simulink model "friction_rt_online_generated"  (R2025a)
settings: Solver=VariableStepAuto  StartTime=0.0  StopTime=100  RelTol=1e-3
settings Model: Creator=Kylo_Ren  LastModifiedBy=Kylo_Ren

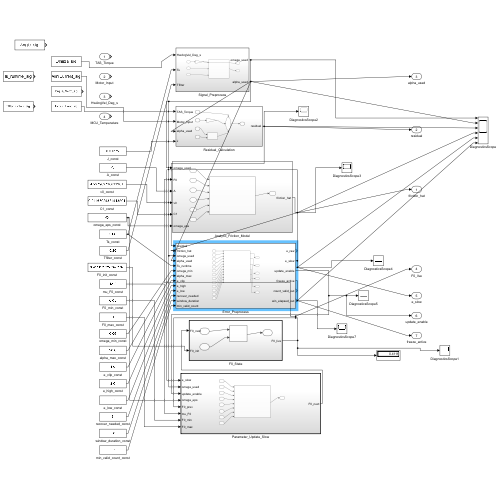
[thumbnail: Simulink's stored preview of the top-level diagram]
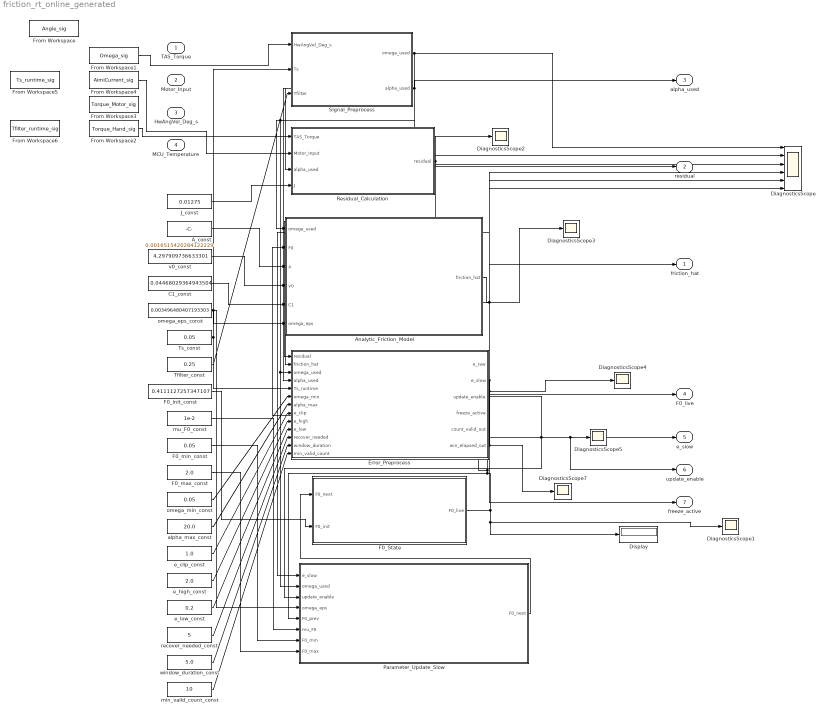
== system friction_rt_online_generated ==
  TAS_Torque : Inport
  Motor_Input : Inport  Port=2
  HwAngVel_Deg_s : Inport  Port=3
  MCU_Temperature : Inport  Port=4
  A_const : Constant  Value=0.0016515420284122229
  Analytic_Friction_Model : Subsystem
  C1_const : Constant  Value=0.04468029364943504
  DiagnosticsScope : Scope  NumInputPorts=6
  DiagnosticsScope{1..5,7} (6 alike) : Scope
      DiagnosticsScope1 settings: ActiveDisplayYMinimum=0.31111272573471072  ActiveDisplayYMaximum=0.51111272573471067
      DiagnosticsScope2 settings: ActiveDisplayYMinimum=-1.2927992978331837  ActiveDisplayYMaximum=1.3052950610427259
      DiagnosticsScope3 settings: ActiveDisplayYMinimum=-0.552517030526273  ActiveDisplayYMaximum=0.552517030526273
      DiagnosticsScope4 settings: ActiveDisplayYMinimum=-1  ActiveDisplayYMaximum=1
      DiagnosticsScope5 settings: ActiveDisplayYMinimum=-1  ActiveDisplayYMaximum=1
      DiagnosticsScope7 settings: ActiveDisplayYMinimum=-1  ActiveDisplayYMaximum=1
  Display : Display
  Error_Preprocess : Subsystem
  F0_State : Subsystem  TreatAsAtomicUnit=on
  F0_init_const : Constant  Value=0.4111127257347107
  F0_max_const : Constant  Value=2.0
  F0_min_const : Constant  Value=0.05
  From Workspace : FromWorkspace  VariableName=Angle_sig
  From Workspace1 : FromWorkspace  VariableName=Omega_sig
  From Workspace2 : FromWorkspace  VariableName=Torque_Hand_sig
  From Workspace3 : FromWorkspace  VariableName=Torque_Motor_sig
  From Workspace4 : FromWorkspace  VariableName=AimiCurrent_sig
  From Workspace5 : FromWorkspace  VariableName=Ts_runtime_sig
  From Workspace6 : FromWorkspace  VariableName=Tfilter_runtime_sig
  J_const : Constant  Value=0.01275
  Parameter_Update_Slow : Subsystem  TreatAsAtomicUnit=on
  Residual_Calculation : Subsystem
  Signal_Preprocess : Subsystem
  Tfilter_const : Constant  Value=0.25
  Ts_const : Constant  Value=0.05
  alpha_max_const : Constant  Value=20.0
  e_clip_const : Constant  Value=1.0
  e_high_const : Constant  Value=2.0
  e_low_const : Constant  Value=0.2
  min_valid_count_const : Constant  Value=10
  mu_F0_const : Constant  Value=1e-2
  omega_eps_const : Constant  Value=0.003496480407193303
  omega_min_const : Constant  Value=0.05
  recover_needed_const : Constant  Value=5
  v0_const : Constant  Value=4.297909736633301
  window_duration_const : Constant  Value=5.0
  friction_hat : Outport
  residual : Outport  Port=2
  alpha_used : Outport  Port=3
  F0_live : Outport  Port=4
  e_slow : Outport  Port=5
  update_enable : Outport  Port=6
  freeze_active : Outport  Port=7
  wires:
  From Workspace1/1 -> Signal_Preprocess/1(HwAngVel_Deg_s)
  Ts_const/1 -> Signal_Preprocess/2(Ts), Error_Preprocess/5(Ts_runtime)
  Tfilter_const/1 -> Signal_Preprocess/3(Tfilter)
  Signal_Preprocess/1(omega_used) -> Error_Preprocess/3(omega_used), Parameter_Update_Slow/2(omega_used), Analytic_Friction_Model/1(omega_used), DiagnosticsScope/1
  Signal_Preprocess/2(alpha_used) -> Residual_Calculation/3(alpha_used), Error_Preprocess/4(alpha_used), alpha_used/1, DiagnosticsScope/2
  From Workspace2/1 -> Residual_Calculation/1(TAS_Torque)
  From Workspace4/1 -> Residual_Calculation/2(Motor_Input)
  J_const/1 -> Residual_Calculation/4(J)
  Residual_Calculation/1(residual) -> Error_Preprocess/1(residual), residual/1, DiagnosticsScope/3, DiagnosticsScope2/1
  Analytic_Friction_Model/1(friction_hat) -> Error_Preprocess/2(friction_hat), friction_hat/1, DiagnosticsScope/4, DiagnosticsScope3/1
  omega_min_const/1 -> Error_Preprocess/6(omega_min)
  alpha_max_const/1 -> Error_Preprocess/7(alpha_max)
  e_clip_const/1 -> Error_Preprocess/8(e_clip)
  e_high_const/1 -> Error_Preprocess/9(e_high)
  e_low_const/1 -> Error_Preprocess/10(e_low)
  recover_needed_const/1 -> Error_Preprocess/11(recover_needed)
  window_duration_const/1 -> Error_Preprocess/12(window_duration)
  min_valid_count_const/1 -> Error_Preprocess/13(min_valid_count)
  Error_Preprocess/2(e_slow) -> e_slow/1, DiagnosticsScope/5, DiagnosticsScope4/1, Parameter_Update_Slow/1(e_slow)
  Error_Preprocess/3(update_enable) -> update_enable/1, DiagnosticsScope5/1, Parameter_Update_Slow/3(update_enable)
  omega_eps_const/1 -> Parameter_Update_Slow/4(omega_eps), Analytic_Friction_Model/6(omega_eps)
  F0_State/1(F0_live) -> DiagnosticsScope1/1, Display/1, Parameter_Update_Slow/5(F0_prev), Analytic_Friction_Model/2(F0), F0_live/1
  mu_F0_const/1 -> Parameter_Update_Slow/6(mu_F0)
  F0_min_const/1 -> Parameter_Update_Slow/7(F0_min)
  F0_max_const/1 -> Parameter_Update_Slow/8(F0_max)
  Parameter_Update_Slow/1(F0_next) -> F0_State/1(F0_next)
  F0_init_const/1 -> F0_State/2(F0_init)
  A_const/1 -> Analytic_Friction_Model/3(A)
  v0_const/1 -> Analytic_Friction_Model/4(v0)
  C1_const/1 -> Analytic_Friction_Model/5(C1)
  Error_Preprocess/4(freeze_active) -> freeze_active/1, DiagnosticsScope/6, DiagnosticsScope7/1

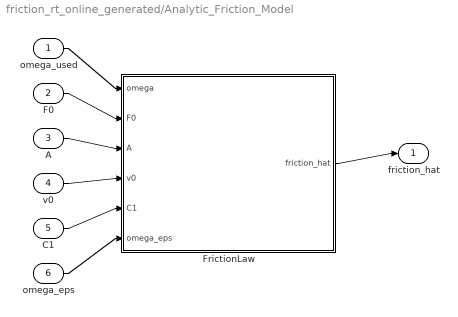
== system friction_rt_online_generated/Analytic_Friction_Model ==
  omega_used : Inport
  F0 : Inport  Port=2
  A : Inport  Port=3
  v0 : Inport  Port=4
  C1 : Inport  Port=5
  omega_eps : Inport  Port=6
  FrictionLaw : MATLAB Function  TreatAsAtomicUnit=on
  friction_hat : Outport
  wires:
  omega_used/1 -> FrictionLaw/1(omega)
  F0/1 -> FrictionLaw/2(F0)
  A/1 -> FrictionLaw/3(A)
  v0/1 -> FrictionLaw/4(v0)
  C1/1 -> FrictionLaw/5(C1)
  omega_eps/1 -> FrictionLaw/6(omega_eps)
  FrictionLaw/1(friction_hat) -> friction_hat/1

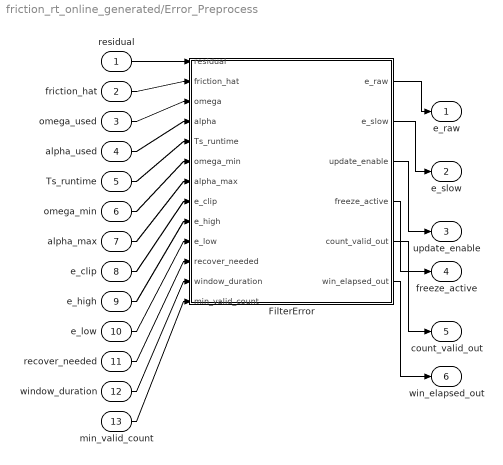
== system friction_rt_online_generated/Error_Preprocess ==
  residual : Inport
  friction_hat : Inport  Port=2
  omega_used : Inport  Port=3
  alpha_used : Inport  Port=4
  Ts_runtime : Inport  Port=5
  omega_min : Inport  Port=6
  alpha_max : Inport  Port=7
  e_clip : Inport  Port=8
  e_high : Inport  Port=9
  e_low : Inport  Port=10
  recover_needed : Inport  Port=11
  window_duration : Inport  Port=12
  min_valid_count : Inport  Port=13
  FilterError : MATLAB Function  TreatAsAtomicUnit=on
  e_raw : Outport
  e_slow : Outport  Port=2
  update_enable : Outport  Port=3
  freeze_active : Outport  Port=4
  count_valid_out : Outport  Port=5
  win_elapsed_out : Outport  Port=6
  wires:
  residual/1 -> FilterError/1(residual)
  friction_hat/1 -> FilterError/2(friction_hat)
  omega_used/1 -> FilterError/3(omega)
  alpha_used/1 -> FilterError/4(alpha)
  Ts_runtime/1 -> FilterError/5(Ts_runtime)
  omega_min/1 -> FilterError/6(omega_min)
  alpha_max/1 -> FilterError/7(alpha_max)
  e_clip/1 -> FilterError/8(e_clip)
  e_high/1 -> FilterError/9(e_high)
  e_low/1 -> FilterError/10(e_low)
  recover_needed/1 -> FilterError/11(recover_needed)
  window_duration/1 -> FilterError/12(window_duration)
  min_valid_count/1 -> FilterError/13(min_valid_count)
  FilterError/1(e_raw) -> e_raw/1
  FilterError/2(e_slow) -> e_slow/1
  FilterError/3(update_enable) -> update_enable/1
  FilterError/4(freeze_active) -> freeze_active/1
  FilterError/5(count_valid_out) -> count_valid_out/1
  FilterError/6(win_elapsed_out) -> win_elapsed_out/1

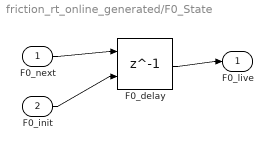
== system friction_rt_online_generated/F0_State ==
  F0_next : Inport
  F0_init : Inport  Port=2
  F0_delay : Delay  DelayLength=1  InitialConditionSource=Input port
      settings: InputPortMap=u0,p4
  F0_live : Outport
  wires:
  F0_next/1 -> F0_delay/1
  F0_init/1 -> F0_delay/2
  F0_delay/1 -> F0_live/1

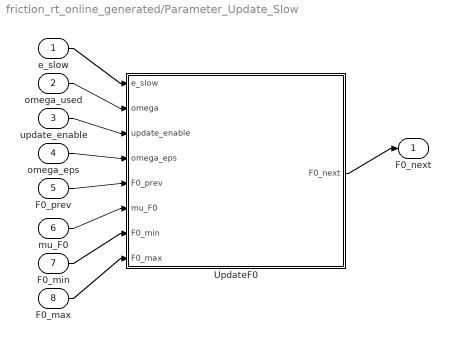
== system friction_rt_online_generated/Parameter_Update_Slow ==
  e_slow : Inport
  omega_used : Inport  Port=2
  update_enable : Inport  Port=3
  omega_eps : Inport  Port=4
  F0_prev : Inport  Port=5
  mu_F0 : Inport  Port=6
  F0_min : Inport  Port=7
  F0_max : Inport  Port=8
  UpdateF0 : MATLAB Function  TreatAsAtomicUnit=on
  F0_next : Outport
  wires:
  e_slow/1 -> UpdateF0/1(e_slow)
  omega_used/1 -> UpdateF0/2(omega)
  update_enable/1 -> UpdateF0/3(update_enable)
  omega_eps/1 -> UpdateF0/4(omega_eps)
  F0_prev/1 -> UpdateF0/5(F0_prev)
  mu_F0/1 -> UpdateF0/6(mu_F0)
  F0_min/1 -> UpdateF0/7(F0_min)
  F0_max/1 -> UpdateF0/8(F0_max)
  UpdateF0/1(F0_next) -> F0_next/1

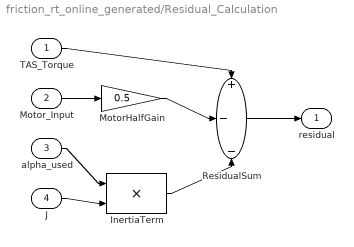
== system friction_rt_online_generated/Residual_Calculation ==
  TAS_Torque : Inport
  Motor_Input : Inport  Port=2
  alpha_used : Inport  Port=3
  J : Inport  Port=4
  InertiaTerm : Product
  MotorHalfGain : Gain  Gain=0.5
  ResidualSum : Sum  Inputs=+--
  residual : Outport
  wires:
  TAS_Torque/1 -> ResidualSum/1
  Motor_Input/1 -> MotorHalfGain/1
  MotorHalfGain/1 -> ResidualSum/2
  alpha_used/1 -> InertiaTerm/1
  J/1 -> InertiaTerm/2
  InertiaTerm/1 -> ResidualSum/3
  ResidualSum/1 -> residual/1

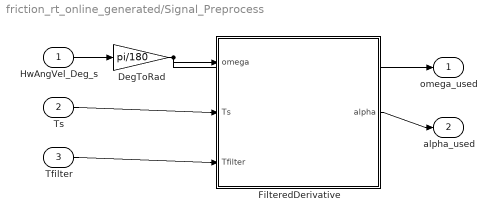
== system friction_rt_online_generated/Signal_Preprocess ==
  HwAngVel_Deg_s : Inport
  Ts : Inport  Port=2
  Tfilter : Inport  Port=3
  DegToRad : Gain  Gain=pi/180
  FilteredDerivative : MATLAB Function  TreatAsAtomicUnit=on
  omega_used : Outport
  alpha_used : Outport  Port=2
  wires:
  HwAngVel_Deg_s/1 -> DegToRad/1
  DegToRad/1 -> FilteredDerivative/1(omega), omega_used/1
  Ts/1 -> FilteredDerivative/2(Ts)
  Tfilter/1 -> FilteredDerivative/3(Tfilter)
  FilteredDerivative/1(alpha) -> alpha_used/1

== matlab function friction_rt_online_generated/Analytic_Friction_Model/FrictionLaw ==
  data: omega input; friction_hat output; F0 input; A input; v0 input; C1 input; omega_eps input
function friction_hat = fcn(omega, F0, A, v0, C1, omega_eps)                             
                                                                                        % Analytic friction law:                                                                 
                                                                                        % friction_hat = tanh(omega/omega_eps) * (F0 + A*(1-exp(-abs(omega)/v0)) + C1*abs(omega))
                                                                                        absw = abs(omega);                                                                       
                                                                                        s = tanh(omega / max(omega_eps, 1e-6));                                                  
                                                                                        phi = 1.0 - exp(-absw / max(v0, 1e-6));                                                  
                                                                                        mag = F0 + A * phi + C1 * absw;                                                          
                                                                                        if mag < 0.0                                                                             
                                                                                            mag = 0.0;                                                                           
                                                                                        end                                                                                      
                                                                                        friction_hat = s * mag;

== matlab function friction_rt_online_generated/Signal_Preprocess/FilteredDerivative ==
  data: omega input; alpha output; Ts input; Tfilter input
function alpha = fcn(omega, Ts, Tfilter)        
                                               % Filtered derivative used for the inertia term.
                                               % X[k] = (Ts/T) * omega[k] + (1 - Ts/T) * X[k-1]
                                               % alpha[k] = (1/T) * (omega[k] - X[k-1])        
                                               persistent x_prev                               
                                               if isempty(x_prev)                              
                                                   x_prev = omega;                             
                                               end                                             
                                               a = Ts / max(Tfilter, 1e-6);                    
                                               a = min(max(a, 0.0), 1.0);                      
                                               alpha = (omega - x_prev) / max(Tfilter, 1e-6);  
                                               x_new = a * omega + (1.0 - a) * x_prev;         
                                               x_prev = x_new;

== matlab function friction_rt_online_generated/Error_Preprocess/FilterError ==
  data: residual input; e_raw output; friction_hat input; omega input; alpha input; Ts_runtime input; omega_min input; alpha_max input; e_clip input; e_high input; e_low input; recover_needed input; window_duration input; min_valid_count input; e_slow output; update_enable output; freeze_active output; count_valid_out output; win_elapsed_out output
function [e_raw, e_slow, update_enable, freeze_active, count_valid_out, win_elapsed_out] = fcn(residual, friction_hat, omega, alpha, Ts_runtime, omega_min, alpha_max, e_clip, e_high, e_low, recover_needed, window_duration, min_valid_count)
    % Build a reliable batch adaptation error.                                                                                                                                                                   
    % 1) compute signed mismatch e_raw for diagnostics                                                                                                                                                           
    % 2) compute magnitude-domain mismatch for F0 adaptation                                                                                                                                                     
    % 3) collect trusted samples in a time window                                                                                                                                                                
    % 4) update only once per window using the window average                                                                                                                                                    
    persistent e_hold freeze_state recover_count win_elapsed sum_mag count_valid                                                                                                                                 
    if isempty(e_hold)                                                                                                                                                                                           
    e_hold = 0.0;                                                                                                                                                                                            
    freeze_state = false;                                                                                                                                                                                    
    recover_count = 0;                                                                                                                                                                                       
    win_elapsed = 0.0;                                                                                                                                                                                       
    sum_mag = 0.0;                                                                                                                                                                                           
    count_valid = 0;                                                                                                                                                                                         
    end                                                                                                                                                                                                          
    e_raw = residual - friction_hat;                                                                                                                                                                             
    e_mag = abs(residual) - abs(friction_hat);                                                                                                                                                                   
    trusted_sample = (abs(omega) > omega_min) && (abs(alpha) < alpha_max);                                                                                                                                       
    anomaly = (abs(e_raw) > e_high) || (abs(alpha) > alpha_max);                                                                                                                                                 
    recovered = trusted_sample && (abs(e_raw) < e_low);                                                                                                                                                          
    if ~freeze_state && anomaly                                                                                                                                                                                  
    freeze_state = true;                                                                                                                                                                                     
    recover_count = 0;                                                                                                                                                                                       
    elseif freeze_state                                                                                                                                                                                          
    if recovered                                                                                                                                                                                             
    recover_count = recover_count + 1;                                                                                                                                                                   
    if recover_count >= recover_needed                                                                                                                                                                   
    freeze_state = false;                                                                                                                                                                            
    recover_count = 0;                                                                                                                                                                               
    end                                                                                                                                                                                                  
    else                                                                                                                                                                                                     
    recover_count = 0;                                                                                                                                                                                   
    end                                                                                                                                                                                                      
    end                                                                                                                                                                                                          
    freeze_active = freeze_state;                                                                                                                                                                                
    sample_ok = trusted_sample && ~freeze_state;                                                                                                                                                                 
    e_used = e_mag;                                                                                                                                                                                              
    if e_used > e_clip                                                                                                                                                                                           
    e_used = e_clip;                                                                                                                                                                                         
    elseif e_used < -e_clip                                                                                                                                                                                      
    e_used = -e_clip;                                                                                                                                                                                        
    end                                                                                                                                                                                                          
    update_enable = false;                                                                                                                                                                                       
    win_elapsed = win_elapsed + max(Ts_runtime, 0.0);                                                                                                                                                            
    if sample_ok                                                                                                                                                                                                 
    sum_mag = sum_mag + e_used;                                                                                                                                                                              
    count_valid = count_valid + 1;                                                                                                                                                                           
    end                                                                                                                                                                                                          
    if win_elapsed >= max(window_duration, max(Ts_runtime, 1e-6))                                                                                                                                                
    if count_valid >= max(1, round(min_valid_count))                                                                                                                                                         
    e_hold = sum_mag / count_valid;                                                                                                                                                                      
    update_enable = true;                                                                                                                                                                                
    end                                                                                                                                                                                                      
    win_elapsed = 0.0;                                                                                                                                                                                       
    sum_mag = 0.0;                                                                                                                                                                                           
    count_valid = 0;                                                                                                                                                                                         
    end                                                                                                                                                                                                          
    e_slow = e_hold;         
    count_valid_out = count_valid;
    win_elapsed_out = win_elapsed;

== matlab function friction_rt_online_generated/Parameter_Update_Slow/UpdateF0 ==
  data: e_slow input; F0_next output; omega input; update_enable input; omega_eps input; F0_prev input; mu_F0 input; F0_min input; F0_max input
function F0_next = fcn(e_slow, omega, update_enable, omega_eps, F0_prev, mu_F0, F0_min, F0_max)
                                                                                              % Batch F0 adaptation using a windowed magnitude-domain error.                                 
                                                                                              % F0 is a magnitude baseline, so the update does not depend on omega sign.                     
                                                                                              F0_next = F0_prev;                                                                             
                                                                                              if update_enable                                                                               
                                                                                                  F0_next = F0_prev + mu_F0 * e_slow;                                                        
                                                                                              end                                                                                            
                                                                                              if F0_next < F0_min                                                                            
                                                                                                  F0_next = F0_min;                                                                          
                                                                                              elseif F0_next > F0_max                                                                        
                                                                                                  F0_next = F0_max;                                                                          
                                                                                              end
